simulink model "GeschlossenerRegelkreis3"  (Simulink 9.3)
settings: Solver=ode45  StartTime=0.0  StopTime=10.0  MaxStep=1e-3  RelTol=1e-3
values from neighbouring files (symbols this model uses):
  h_matrix = inv(A) * (phi_matrix - eye(size(phi_matrix,1))) * B    [A3Main.m]
  K_M = 1/63000    (= 1.5873015873e-05)    [A3Main.m]
  phi_matrix = expm(A * T_a)    [A3Main.m]
  T_a = 0.015    [A3Main.m]
  U_step = 0.5    [A3Main.m]
undefined symbols (not defined in the file or in its folder): C, D, DiscIntNeverNeededParam
settings Model: Creator=wredi  LastModifiedBy=wredi
settings DataIOCC: SaveFormat=Dataset  SignalLoggingSaveFormat=Dataset  ReturnWorkspaceOutputs=on
settings DebuggingCC: UnderspecifiedInitializationDetection=Simplified  MergeDetectMultiDrivingBlocksExec=error  FcnCallInpInsideContextMsg=error  SFUnexpectedBacktrackingDiag=error  SFNoUnconditionalDefaultTransitionDiag=error  SFExecutionAtInitializationDiag=warning
settings HardwareCC: ProdBitPerPointer=64  ProdBitPerSizeT=64  ProdBitPerPtrDiffT=64  ProdLargestAtomicFloat=Float  ProdIntDivRoundTo=Zero  ProdEndianess=LittleEndian  ProdWordSize=64  ProdHWDeviceType=Intel->x86-64 (Windows64)
settings ModelReferenceCC: PropagateSignalLabelsOutOfModel=on
settings SFSimCC: SimUseLocalCustomCode=on
settings RTWCC: RTWUseLocalCustomCode=on
settings CodeAppCC: StateflowObjectComments=off
settings GRTTargetCC: TargetLangStandard=C99 (ISO)  CombineOutputUpdateFcns=on  GRTInterface=off
settings ConfigComp: CovMetricSettings=dwe  CovHtmlReporting=off  CovSaveCumulativeToWorkspaceVar=off  CovSaveSingleToWorkspaceVar=off  CovExternalEMLEnable=on

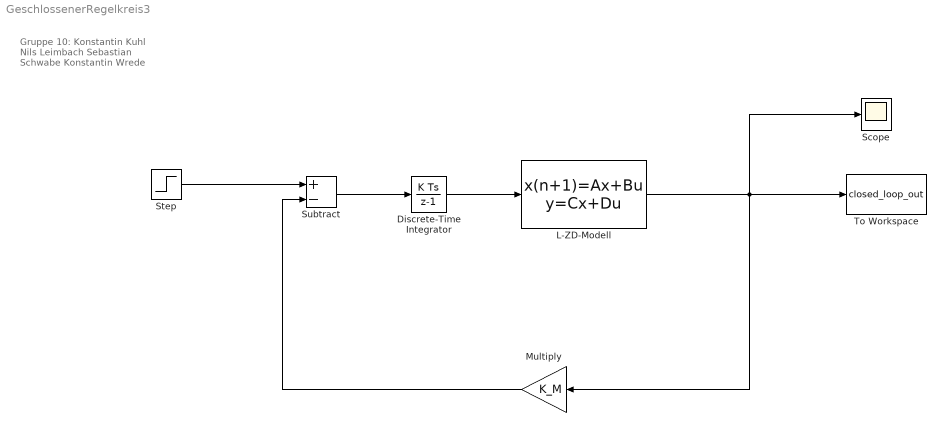
== system GeschlossenerRegelkreis3 ==
  note: Gruppe 10:
      | Konstantin Kuhl
      | Nils Leimbach
      | Sebastian Schwabe
      | Konstantin Wrede
  Discrete-Time Integrator : DiscreteIntegrator  gainval=K_I_controller  SampleTime=T_a  ICPrevOutput=DiscIntNeverNeededParam  ICPrevScaledInput=DiscIntNeverNeededParam
  L-ZD-Modell : DiscreteStateSpace  A=phi_matrix  B=h_matrix  C=C  D=D  SampleTime=T_a
  Multiply : Gain  Gain=K_M
  Scope : Scope
  Step : Step  After=U_step  SampleTime=0
  Subtract : Sum  Inputs=+-
  To Workspace : ToWorkspace  VariableName=closed_loop_out  SaveFormat=Structure With Time  SampleTime=-1
  wires:
  Discrete-Time Integrator/1 -> L-ZD-Modell/1
  L-ZD-Modell/1 -> Multiply/1, To Workspace/1, Scope/1
  Multiply/1 -> Subtract/2
  Subtract/1 -> Discrete-Time Integrator/1
  Step/1 -> Subtract/1
